simulink model "ControlledMotion"  (R2024a)
settings: Solver=VariableStepAuto  StartTime=0.0  StopTime=tspan  FixedStep=10  RelTol=1e-3
model workspace: external: MAT-File /Users/bricenrigby/Documents/Poly Sim/SACS Program/Dynamics Simulations Testing/Simulink Modeling/ControlledMotionScript.mat (data not in the file)
values from neighbouring files (symbols this model uses):
  dOff = 0.1    [ControlledMotionScript.m]
  dOn = 0.15    [ControlledMotionScript.m]
  J = [0.096 0 0; 0 0.096 0; 0 0 0.166]    [ControlledMotionScript.m]    (also in TorqueFreeMotionScript.m = [0.016 0 0; 0 0.016 0; 0 0 0.025])
  Kd = .02    (= 0.02)    [ControlledMotionScript.m]
  Kp = .010    (= 0.01)    [ControlledMotionScript.m]
  theta_b_0 = [0;0;180]    [ControlledMotionScript.m]
  thrust = 0.312 * 1 * 4    (= 1.248)    [ControlledMotionScript.m]
  w_b_0 = [0.000; 0.000; 0.000]    [ControlledMotionScript.m]    (also in TorqueFreeMotionScript.m)
settings Model: Creator=emehiel  LastModifiedBy=bricenrigby
settings SolverCC: AlgebraicLoopSolver=TrustRegion
settings OptimizationCC: ReuseModelBlockBuffer=off
settings DebuggingCC: UnconnectedInputMsg=warning  UnconnectedOutputMsg=warning  UnconnectedLineMsg=warning  UnderSpecifiedDimensionMsg=warning
settings ModelReferenceCC: EnableRefExpFcnMdlSchedulingChecks=on
settings RTWCC: GPUComputeCapability=3.5

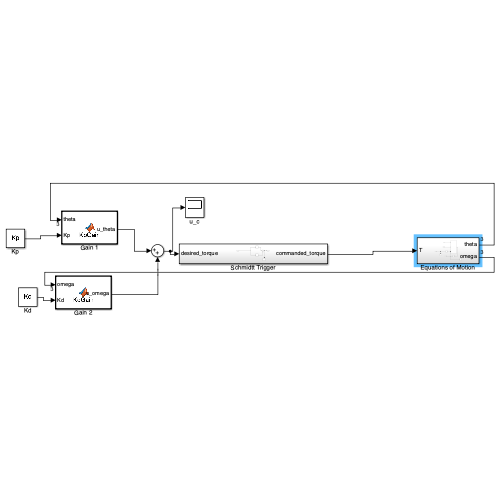
[thumbnail: Simulink's stored preview of the top-level diagram]
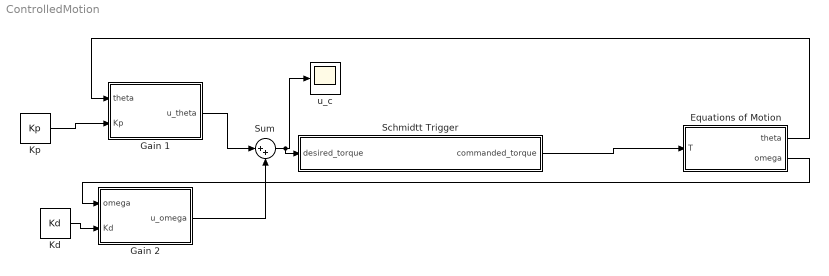
== system ControlledMotion ==
  Equations of Motion : Subsystem
  Gain 1 : MATLAB Function  TreatAsAtomicUnit=on
  Gain 2 : MATLAB Function  TreatAsAtomicUnit=on
  Kd : Constant  Value=Kd
  Kp : Constant  Value=Kp
  Schmidtt Trigger : Subsystem
  Sum : Sum  Inputs=|++
  u_c : Scope
  wires:
  Gain 1/1(u_theta) -> Sum/1
  Equations of Motion/1(theta) -> Gain 1/1(theta)
  Equations of Motion/2(omega) -> Gain 2/1(omega)
  Gain 2/1(u_omega) -> Sum/2
  Sum/1 -> u_c/1, Schmidtt Trigger/1(desired_torque)
  Schmidtt Trigger/1(commanded_torque) -> Equations of Motion/1(T)
  Kp/1 -> Gain 1/2(Kp)
  Kd/1 -> Gain 2/2(Kd)

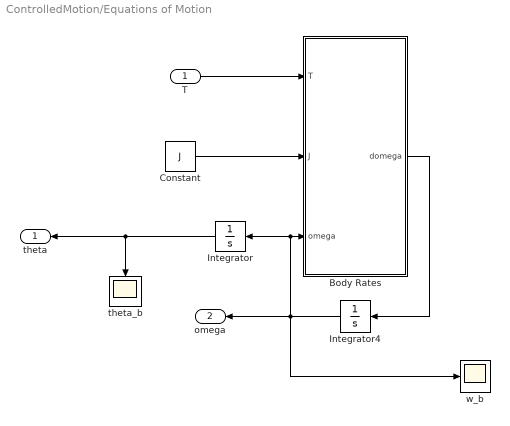
== system ControlledMotion/Equations of Motion ==
  T : Inport
  Body Rates : MATLAB Function  TreatAsAtomicUnit=on
  Constant : Constant  Value=J
  Integrator : Integrator  InitialCondition=theta_b_0
  Integrator4 : Integrator  InitialCondition=w_b_0
  theta_b : Scope
  w_b : Scope
  theta : Outport
  omega : Outport  Port=2
  wires:
  Body Rates/1(domega) -> Integrator4/1
  Integrator4/1 -> Integrator/1, Body Rates/3(omega), omega/1, w_b/1
  T/1 -> Body Rates/1(T)
  Integrator/1 -> theta_b/1, theta/1
  Constant/1 -> Body Rates/2(J)

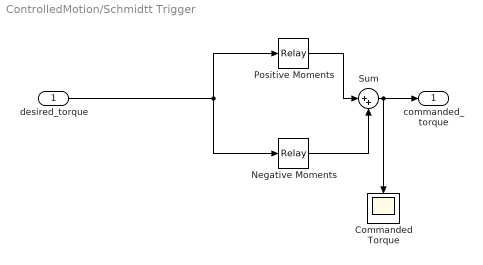
== system ControlledMotion/Schmidtt Trigger ==
  desired_torque : Inport
  Commanded Torque : Scope
  Negative Moments : Relay  OnSwitchValue=dOff  OffSwitchValue=-dOn  OnOutputValue=0  OffOutputValue=-thrust
  Positive Moments : Relay  OnSwitchValue=dOn  OffSwitchValue=-dOff  OnOutputValue=thrust
  Sum : Sum  Inputs=|++
  commanded_torque : Outport
  wires:
  Positive Moments/1 -> Sum/1
  Negative Moments/1 -> Sum/2
  desired_torque/1 -> Positive Moments/1, Negative Moments/1
  Sum/1 -> Commanded Torque/1, commanded_torque/1

== matlab function ControlledMotion/Gain 1 ==
  data: theta input; u_theta output; Kp input
function u_theta = KpGain(theta, Kp)
%#codegen

u_theta = -Kp * theta(3);

end

== matlab function ControlledMotion/Gain 2 ==
  data: omega input; u_omega output; Kd input
function u_omega = KdGain(omega, Kd)
%#codegen

u_omega = -Kd * omega(3);

end

== matlab function ControlledMotion/Equations of Motion/Body Rates ==
  data: T input; J input; omega input; domega output
function domega = dynamics(T, J, omega)
%#codegen

% Compute the derivative of the angular velocity $\omega$ here
Ix = J(1,1);
Iy = J(2,2);
Iz = J(3,3);

wdot1 = (0 - (Iz-Iy)*omega(2)*omega(3))/Ix;
wdot2 = (0 - (Ix-Iz)*omega(1)*omega(3))/Iy;
wdot3 = (T - (Iy-Ix)*omega(1)*omega(2))/Iz;

domega = [wdot1; wdot2; wdot3];

end
